simulink model "model_main4"  (R2023b)
settings: Solver=ode4  StartTime=0.0  StopTime=1000  FixedStep=dt  RelTol=1e-3
values from neighbouring files (symbols this model uses):
  dt = 0.01    [model_init.m]
  Iws = diag([1 1 1 1])*0.227    [model_init.m]
  m_tot = 3019.19    [model_init.m]
  Omega1_init = 1000*rpm2rad    (= 104.71975512)    [model_init.m]
  Omega2_init = 1000*rpm2rad    (= 104.71975512)    [model_init.m]
  Omega3_init = 1000*rpm2rad    (= 104.71975512)    [model_init.m]
  Omega4_init = 1000*rpm2rad    (= 104.71975512)    [model_init.m]
  qb0 = eul2quat(ag0','ZYX')'    [model_init.m]
  rad2rpm = 1/rpm2rad    (= 9.54929658551)    [model_init.m]
  RCS_F = 1.0    (= 1)    [model_init.m]
  RCS_Pos = [RCS1_POS , RCS2_POS , RCS3_POS , RCS4_POS ,            RCS5_POS , RCS6_POS , RCS7_POS , RCS8_POS ,            RCS9_POS , RCS10_POS, RCS11_POS, RCS12_POS,            RCS13_POS, RCS14_POS, RCS15_POS, RCS16_POS]    [model_init.m]
  RCS_PWM_Freq = 0.5    [model_init.m]
  RCS_Sampling_time = 0.01    [model_init.m]
  RCS_THR_vec = [RCS1_THR , RCS2_THR , RCS3_THR , RCS4_THR,                 RCS5_THR , RCS6_THR , RCS7_THR , RCS8_THR,                 RCS9_THR , RCS10_THR, RCS11_THR, RCS12_THR,                 RCS13_THR, RCS14_THR, RCS15_THR, RCS16_THR]    [model_init.m]
  REL_TS_POS_I_0 = TS_pos0 - SC_pos0    [model_init.m]
  REL_TS_VEL_I_0 = TS_vel0 - SC_vel0    [model_init.m]
  RW_As = [RW1_Axis,RW2_Axis,RW3_Axis,RW4_Axis]    [model_init.m]
  RW_Omegad_max = 4200*rpm2rad    (= 439.822971503)    [model_init.m]
  SC_Ib = [1257.52 -0.07285  -0.0345 ... (first row only)    [model_init.m]
  SC_state0 = kepel_statvec (SC_Kepler)    [model_init.m]
  TS_Ib = diag([1 1 1])    [model_init.m]
  TS_qb0 = angle2quat(deg2rad(0),deg2rad(0),deg2rad(0),'ZYX')'    [model_init.m]
  TS_state0 = kepel_statvec (TS_Kepler)    [model_init.m]
  TS_wb0 = deg2rad([0 0 0]')    [model_init.m]
  wb0 = [0 0 0]'    [model_init.m]
undefined symbols (not defined in the file or in its folder): norm_Ib, RCS_F_vec, RCS_pos, RW_Max_Speed, SS_Total_Mass, TC_Kepler
libraries: simulink x16, simulink_extras x13, sharedtransform x9, aerolibutil x8
(part 1 of 2)
settings Model: PacingRate=1.100000  Creator=yhj2019  LastModifiedBy=ASCL
settings DebuggingCC: UnderSpecifiedDimensionMsg=warning

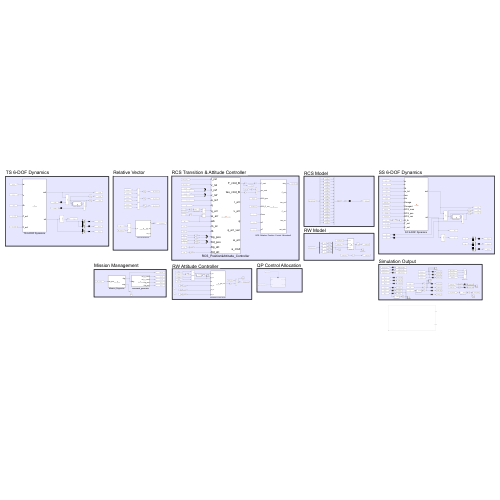
[thumbnail: Simulink's stored preview of the top-level diagram]
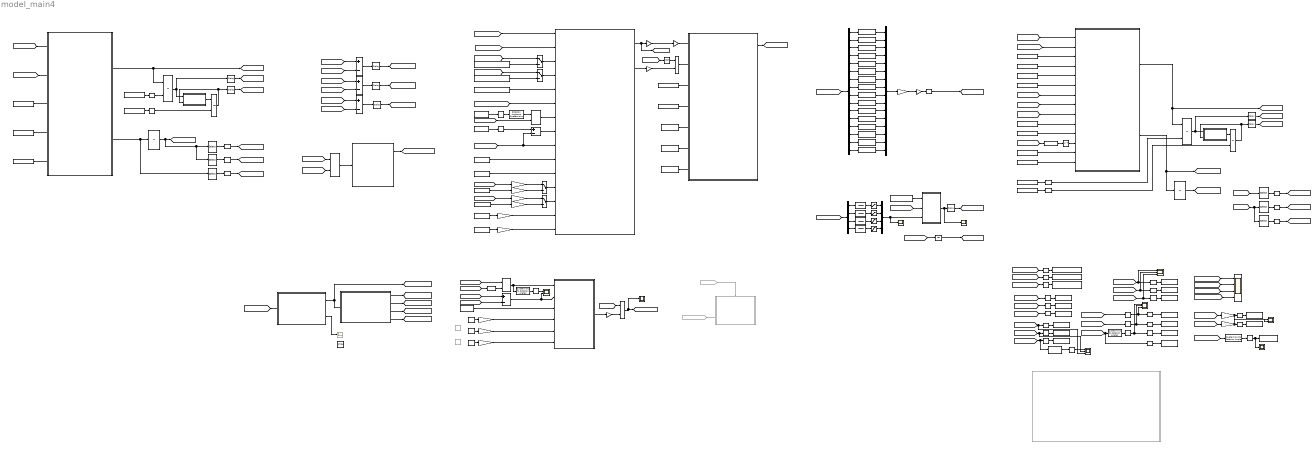
== system model_main4 ==
  note: TS 6-DOF Dynamics
  note: RW Model
  note: RW Attitude Controller
  note: RCS Model
  note: Simulation Output
  note: RCS Transition & Attitude Controller
  note: SS 6-DOF Dynamics
  note: Relative Vector
  note: Mission Management
  note: QP Control Allocation
  Add{,1..3,10} (5 alike) : Sum  Inputs=+-
  Constant : Constant  Value=0.3
  Constant1 : Constant  Value=17
  Constant{7,10,15,23,39,52} (6 alike) : Constant  Value=[0 0 0]'
  Constant11 : Constant  Value=RCS_Pos
  Constant12 : Constant  Value=RCS_THR_vec
  Constant13 : Constant  Value=m_tot
  Constant14 : Constant  Value=RW_Max_Speed
  Constant16 : Constant  Commented=on  Value=20
  Constant17 : Constant  Commented=on  Value=1000
  Constant18 : Constant  Value=200
  Constant19 : Constant  Value=10000
  Constant2 : Constant  Value=200
  Constant20 : Constant  Value=m_tot
  Constant21 : Constant  Value=0
  Constant3 : Constant  Value=2000
  Constant32 : Constant  Value=RW_As
  Constant36 : Constant  Value=TS_Ib
  Constant4 : Constant  Value=SC_Ib
  Constant40 : Constant  Value=TS_wb0
  Constant41 : Constant  Value=TS_qb0
  Constant49 : Constant  Value=[5.0 0 0]'
  Constant5 : Constant  Value=Iws
  Constant53 : Constant  Value=SC_Ib
  Constant55 : Constant
  Constant56 : Constant  Value=0.5
  Constant57 : Constant  Value=0.5
  Constant58 : Constant  Value=[0 0 0]
  Constant59 : Constant  Value=[0 0 0]
  Constant6 : Constant  Value=RW_As
  Constant60 : Constant  Value=RCS_Pos
  Constant61 : Constant  Value=RCS_THR_vec
  Constant8 : Constant  Value=wb0
  Constant9 : Constant  Value=qb0
  Degrees to Radians2 : simulink_extras/Transformations/Degrees to Radians
  Degrees to Radians3 : simulink_extras/Transformations/Degrees to Radians
  Demux : Demux  Outputs=16
  Demux1 : Demux
  Enabled Subsystem : Subsystem  Commented=on  TreatAsAtomicUnit=on
  From33 : From  Commented=on  GotoTag=mission_flag  TagVisibility=global
  From39 : From  Commented=on  GotoTag=RW_torque_cmd
  Gain{1,3,5..7,9,13,18,20} (9 alike) : Gain  Gain=norm_Ib
  Gain{2,10,12,23} (4 alike) : Gain
  Gain11 : Gain  Gain=rad2rpm
  Gain22 : Gain  Gain=-1
  Gain4 : Gain  Gain=RCS_F
  Gain8 : Gain  Gain=rad2rpm
  Get LOS Quaternion : MATLAB Function  TreatAsAtomicUnit=on
  Inetial to body : aerolibutil/Quaternion Rotation
  Integrator : Integrator  InitialConditionSource=external  InitialCondition=wb0
  Integrator2 : Integrator  InitialConditionSource=external  InitialCondition=wb0
  Integrator3 : Integrator  InitialCondition=[Omega1_init Omega2_init Omega3_init Omega4_init]'
  Integrator4 : Integrator  InitialConditionSource=external
  Integrator5 : Integrator  InitialCondition=TS_state0'
  Integrator7 : Integrator  InitialConditionSource=external
  Integrator8 : Integrator  InitialCondition=SC_state0'
  Los angle : Scope
  Manual Switch{,1,3..4} (4 alike) : ManualSwitch
  Mission_Supporter : MATLAB Function  TreatAsAtomicUnit=on
  Mux1 : Mux
  Mux2 : Mux  Inputs=16
  NOT : Logic  Operator=NOT  IconShape=distinctive  AllPortsSameDT=off  OutDataTypeStr=boolean
  PWM{,1..15} (16 alike) : simulink/Discontinuities/PWM  DisableCoverage=on  Period=RCS_PWM_Freq  InitialDelay=0  DisallowZeroDutyCycle=off  RunAtFixedTimeIntervals=on  SampleTime=RCS_Sampling_time
  Product : Product
  Product1 : Product
  Quaternion Inverse : aerolibutil/Quaternion Inverse
  Quaternion Multiplication1 : aerolibutil/Quaternion Multiplication
  Quaternion Multiplication4 : aerolibutil/Quaternion Multiplication
  Quaternion_Kinematics : MATLAB Function  TreatAsAtomicUnit=on
  Quaternion_Kinematics1 : MATLAB Function  TreatAsAtomicUnit=on
  Quaternions to Direction Cosine Matrix : sharedtransform/Quaternions to  Direction Cosine Matrix  aMode=aMode
      settings: LibrarySourceBlock=|
      | aerolibtransform2/Quaternions to
      | Direction Cosine Matrix
  Quaternions to Rotation Angles{,1..3} (4 alike) : sharedtransform/Quaternions to Rotation Angles  rotationOrder=ZYX  aMode=aMode
  RCS_Position&Attitude_Controller : MATLAB Function  TreatAsAtomicUnit=on
  RCS_Relative_Position_Control_Allocation2 : MATLAB Function  TreatAsAtomicUnit=on
  RW_torque_cmd : Scope
  Radians to Degrees{,1..5} (6 alike) : simulink_extras/Transformations/Radians to Degrees
  Rel transition / flag : Scope  NumInputPorts=4
  Reshape{,1..2,12..14,19..23} (11 alike) : Reshape  OutputDimensionality=Column vector (2-D)
  Reshape{3..11,15..18,24..28} (18 alike) : Reshape  OutputDimensionality=Row vector (2-D)
  Rotation Angles to Quaternions2 : sharedtransform/Rotation Angles to Quaternions  rotationOrder=ZYX  aMode=aMode
  SC 6-DOF Dynamics : MATLAB Function  TreatAsAtomicUnit=on
  SS Attitude Control wrt ECI : MATLAB Function  TreatAsAtomicUnit=on
  SS attitude : Scope  NumInputPorts=3
  SS transition : Scope  NumInputPorts=3
  Saturation{1..4} (4 alike) : Saturate  UpperLimit=RW_Omegad_max  LowerLimit=-RW_Omegad_max
  Scope : Scope  Commented=on
  Scope1 : Scope
  Scope2 : Scope
  Selector1 : Selector  InputPortWidth=6  IndexOptions=Index vector (dialog)  Indices=[1 2 3]  OutputSizes=1
  Selector2 : Selector  InputPortWidth=6  IndexOptions=Index vector (dialog)  Indices=[4 5 6]  OutputSizes=1
  Selector6 : Selector  InputPortWidth=6  IndexOptions=Index vector (dialog)  Indices=[1 2 3]  OutputSizes=1
  Selector7 : Selector  InputPortWidth=6  IndexOptions=Index vector (dialog)  Indices=[1 2 3]  OutputSizes=1
  Selector8 : Selector  InputPortWidth=6  IndexOptions=Index vector (dialog)  Indices=[4 5 6]  OutputSizes=1
  Selector9 : Selector  InputPortWidth=6  IndexOptions=Index vector (dialog)  Indices=[4 5 6]  OutputSizes=1
  Stop Simulation : Stop
  Subsystem : Subsystem  Commented=on
  TS 6-DOF Dynamics : MATLAB Function  TreatAsAtomicUnit=on
  Target attitude : Scope  NumInputPorts=3
  To Workspace : ToWorkspace  VariableName=SS_POS_I  SampleTime=-1
      settings: Save2DSignal=2-D array (concatenate along first dimension)
  To Workspace1 : ToWorkspace  VariableName=SS_VEL_I  SampleTime=-1
      settings: Save2DSignal=2-D array (concatenate along first dimension)
  To Workspace10 : ToWorkspace  VariableName=TS_VEL_I  SampleTime=-1
      settings: Save2DSignal=2-D array (concatenate along first dimension)
  To Workspace11 : ToWorkspace  VariableName=TS_ACC_I  SampleTime=-1
      settings: Save2DSignal=2-D array (concatenate along first dimension)
  To Workspace12 : ToWorkspace  VariableName=SS_q_b  SampleTime=-1
      settings: Save2DSignal=2-D array (concatenate along first dimension)
  To Workspace13 : ToWorkspace  VariableName=TS_wb  SampleTime=-1
      settings: Save2DSignal=2-D array (concatenate along first dimension)
  To Workspace14 : ToWorkspace  VariableName=wheel_rate  SampleTime=-1
      settings: Save2DSignal=2-D array (concatenate along first dimension)
  To Workspace15 : ToWorkspace  VariableName=TS_q  SampleTime=-1
      settings: Save2DSignal=2-D array (concatenate along first dimension)
  To Workspace16 : ToWorkspace  VariableName=TS_wd  SampleTime=-1
      settings: Save2DSignal=2-D array (concatenate along first dimension)
  To Workspace17 : ToWorkspace  VariableName=LoS_angle  SampleTime=-1
      settings: Save2DSignal=2-D array (concatenate along first dimension)
  To Workspace18 : ToWorkspace  VariableName=wheel_rated  SampleTime=-1
      settings: Save2DSignal=2-D array (concatenate along first dimension)
  To Workspace2 : ToWorkspace  VariableName=SS_ACC_I  SampleTime=-1
      settings: Save2DSignal=2-D array (concatenate along first dimension)
  To Workspace3 : ToWorkspace  VariableName=SS_wd_b  SampleTime=-1
      settings: Save2DSignal=2-D array (concatenate along first dimension)
  To Workspace4 : ToWorkspace  VariableName=SS_w_b  SampleTime=-1
      settings: Save2DSignal=2-D array (concatenate along first dimension)
  To Workspace5 : ToWorkspace  VariableName=SS_angle_I  SampleTime=-1
      settings: Save2DSignal=2-D array (concatenate along first dimension)
  To Workspace6 : ToWorkspace  VariableName=REL_TS_POS_I  SampleTime=-1
      settings: Save2DSignal=2-D array (concatenate along first dimension)
  To Workspace7 : ToWorkspace  VariableName=REL_TS_VEL_I  SampleTime=-1
      settings: Save2DSignal=2-D array (concatenate along first dimension)
  To Workspace8 : ToWorkspace  VariableName=REL_TS_ACC_I  SampleTime=-1
      settings: Save2DSignal=2-D array (concatenate along first dimension)
  To Workspace9 : ToWorkspace  VariableName=TS_POS_I  SampleTime=-1
      settings: Save2DSignal=2-D array (concatenate along first dimension)
  Transfer Fcn{,1..3} (4 alike) : TransferFcn  Numerator=[10]  Denominator=[1 10]
  Transport Delay1 : TransportDelay  DelayTime=dt  InitialOutput=qb0
  Transport Delay2 : TransportDelay  DelayTime=dt  InitialOutput=wb0
  Transport Delay3 : TransportDelay  DelayTime=dt  InitialOutput=[0 0 0]'
  Transport Delay4 : TransportDelay  DelayTime=dt  InitialOutput=REL_TS_VEL_I_0
  Transport Delay5 : TransportDelay  DelayTime=dt  InitialOutput=REL_TS_POS_I_0
  Transport Delay6 : TransportDelay  DelayTime=dt  InitialOutput=[0 0 0 0]'
  Transport Delay7 : TransportDelay  DelayTime=dt  InitialOutput=TS_qb0
  Transport Delay8 : TransportDelay  DelayTime=dt  InitialOutput=TS_wb0
  Transpose : Math  Operator=transpose
  attitude error : Scope  NumInputPorts=2
  command_generator : MATLAB Function  TreatAsAtomicUnit=on
  saturation : MATLAB Function  TreatAsAtomicUnit=on
  wheel rate : Scope  NumInputPorts=2
  tag scope: Kd_pos=global, Kp_pos=global, mission_flag=global, rel_p_cmd=global, rel_v_cmd=global
  wires:
  Reshape6/1 -> To Workspace/1
  Reshape7/1 -> To Workspace1/1
  Reshape8/1 -> To Workspace2/1
  [TS_p_I] -> Add/1
  [SS_p_I] -> Add/2
  [SS_v_I] -> Add1/2
  [TS_v_I] -> Add1/1
  [SS_a_I] -> Add2/2
  [TS_a_I] -> Add2/1
  Add/1 -> Transport Delay5/1
  Add1/1 -> Transport Delay4/1
  Add2/1 -> Transport Delay3/1
  Constant4/1 -> SC 6-DOF Dynamics/3(Ib)
  Constant5/1 -> SC 6-DOF Dynamics/5(Iws)
  SC 6-DOF Dynamics/1(wd) -> Integrator/1, [wd]
  [wb] -> SC 6-DOF Dynamics/1(w)
  Constant6/1 -> SC 6-DOF Dynamics/6(As)
  [Omega_mea] -> SC 6-DOF Dynamics/7(Omega)
  [Omegad_mea] -> SC 6-DOF Dynamics/8(Omegad)
  Quaternion_Kinematics/1(qd) -> Integrator7/1
  Constant8/1 -> Reshape19/1
  Constant9/1 -> Reshape20/1
  Quaternions to Rotation Angles/1 -> Radians to Degrees2/1
  [wd] -> Radians to Degrees/1
  [wb] -> Radians to Degrees1/1
  Radians to Degrees/1 -> SS attitude/3, Reshape9/1
  Radians to Degrees1/1 -> SS attitude/2, Reshape10/1
  Radians to Degrees2/1 -> SS attitude/1, Reshape11/1
  [q] -> Reshape3/1, Quaternions to Rotation Angles/1
  Constant10/1 -> SC 6-DOF Dynamics/14(F_ext)
  Constant13/1 -> SC 6-DOF Dynamics/4(m_tot)
  [q] -> Quaternions to Direction Cosine Matrix/1
  Quaternions to Direction Cosine Matrix/1 -> Transpose/1
  [SS_v_I] -> SS transition/2, Reshape7/1
  Transpose/1 -> SC 6-DOF Dynamics/12(R_Ib)
  Reshape9/1 -> To Workspace3/1
  Reshape10/1 -> To Workspace4/1
  Reshape11/1 -> To Workspace5/1
  SC 6-DOF Dynamics/2(xd) -> Integrator8/1, [xd]
  Integrator8/1 -> [x]
  Selector8/1 -> Reshape2/1
  Selector6/1 -> Reshape/1
  [xd] -> Selector8/1, Selector7/1
  [x] -> Selector6/1
  Selector7/1 -> Reshape1/1
  [x] -> SC 6-DOF Dynamics/2(x)
  Constant11/1 -> SC 6-DOF Dynamics/10(RCS_pos)
  Constant12/1 -> SC 6-DOF Dynamics/11(RCS_vec)
  Demux/1 -> PWM/1
  Demux/2 -> PWM1/1
  Demux/3 -> PWM2/1
  Demux/4 -> PWM3/1
  Demux/8 -> PWM7/1
  Demux/5 -> PWM4/1
  Demux/6 -> PWM5/1
  Demux/7 -> PWM6/1
  Demux/14 -> PWM13/1
  Demux/13 -> PWM12/1
  Demux/15 -> PWM14/1
  Demux/12 -> PWM11/1
  Demux/16 -> PWM15/1
  Demux/9 -> PWM8/1
  Demux/10 -> PWM9/1
  Demux/11 -> PWM10/1
  PWM/1 -> Mux2/1
  Mux2/1 -> Gain4/1
  PWM1/1 -> Mux2/2
  PWM2/1 -> Mux2/3
  PWM3/1 -> Mux2/4
  PWM4/1 -> Mux2/5
  PWM5/1 -> Mux2/6
  PWM6/1 -> Mux2/7
  PWM7/1 -> Mux2/8
  PWM8/1 -> Mux2/9
  PWM9/1 -> Mux2/10
  PWM10/1 -> Mux2/11
  PWM11/1 -> Mux2/12
  PWM12/1 -> Mux2/13
  PWM13/1 -> Mux2/14
  PWM14/1 -> Mux2/15
  PWM15/1 -> Mux2/16
  [RCS_mea] -> SC 6-DOF Dynamics/9(RCS_mea)
  Gain4/1 -> Gain12/1
  Reshape/1 -> [SS_p_I]
  Reshape1/1 -> [SS_v_I]
  Reshape2/1 -> [SS_a_I]
  [REL_TS_POS_I] -> Reshape16/1
  [REL_TS_VEL_I] -> Reshape17/1
  [REL_TS_ACC_I] -> Reshape18/1
  Reshape16/1 -> To Workspace6/1
  Reshape17/1 -> To Workspace7/1
  Reshape18/1 -> To Workspace8/1
  [REL_TS_POS_I] -> Rel transition / flag/1
  [REL_TS_VEL_I] -> Rel transition / flag/2
  [REL_TS_ACC_I] -> Rel transition / flag/3
  Constant32/1 -> SS Attitude Control wrt ECI/3(As)
  Get LOS Quaternion/1(q) -> [LoS_Quaternion]  "LOS quaternion"
  Add10/1 -> SS Attitude Control wrt ECI/2(w_err), attitude error/2
  [q] -> Inetial to body/1
  Inetial to body/1 -> Get LOS Quaternion/1(r_rel)
  SS Attitude Control wrt ECI/1(RW_cmd) -> Gain10/1
  [REL_TS_POS_I] -> Inetial to body/2
  Reshape19/1 -> Integrator/2
  Reshape20/1 -> Integrator7/2
  Gain12/1 -> Reshape14/1
  Demux1/1 -> Transfer Fcn/1
  Demux1/4 -> Transfer Fcn3/1
  Demux1/2 -> Transfer Fcn1/1
  Demux1/3 -> Transfer Fcn2/1
  Transfer Fcn/1 -> Saturation4/1
  Transfer Fcn1/1 -> Saturation1/1
  Transfer Fcn2/1 -> Saturation2/1
  Transfer Fcn3/1 -> Saturation3/1
  [Omegad_mea] -> Integrator3/1
  Integrator3/1 -> [Omega_mea]
  Integrator/1 -> Transport Delay2/1, Quaternion_Kinematics/1(w)
  Integrator7/1 -> Transport Delay1/1, Quaternion_Kinematics/2(q)
  [Omegad_mea] -> Gain8/1
  [Omega_mea] -> Gain11/1
  [RW_torque_cmd] -> Demux1/1
  saturation/1(res) -> RW_torque_cmd/1, Transport Delay6/1
  Saturation3/1 -> Mux1/4
  Saturation1/1 -> Mux1/2
  Saturation4/1 -> Mux1/1
  Saturation2/1 -> Mux1/3
  Mux1/1 -> Scope2/1, saturation/3(torque_cmd)
  [Omega_mea] -> saturation/2(Omega_mea)
  Constant14/1 -> saturation/1(max_speed)
  [SS_p_I] -> SS transition/1, Reshape6/1
  [SS_a_I] -> SS transition/3, Reshape8/1
  Reshape14/1 -> [RCS_mea]
  Transport Delay1/1 -> [q]
  Transport Delay2/1 -> [wb]
  Transport Delay3/1 -> [REL_TS_ACC_I]
  Transport Delay4/1 -> [REL_TS_VEL_I]
  Transport Delay5/1 -> [REL_TS_POS_I]
  Transport Delay6/1 -> [Omegad_mea]
  Transport Delay7/1 -> [TS_q]
  Integrator4/1 -> Quaternion_Kinematics1/2(q), Transport Delay7/1
  Constant39/1 -> TS 6-DOF Dynamics/4(T_ext)
  Integrator2/1 -> Quaternion_Kinematics1/1(w), Transport Delay8/1
  Constant41/1 -> Reshape13/1
  Transport Delay8/1 -> [TS_wb]
  Integrator5/1 -> Selector2/1, Selector1/1, [TS_x]
  Reshape13/1 -> Integrator4/2
  TS 6-DOF Dynamics/2(xd) -> Selector9/1, Integrator5/1
  [TS_x] -> TS 6-DOF Dynamics/2(x)
  Quaternion_Kinematics1/1(qd) -> Integrator4/1
  Constant15/1 -> TS 6-DOF Dynamics/5(F_ext)
  TS 6-DOF Dynamics/1(wd) -> [TS_wd], Integrator2/1
  Constant40/1 -> Reshape12/1
  [TS_wb] -> TS 6-DOF Dynamics/1(w)
  Constant36/1 -> TS 6-DOF Dynamics/3(Ib)
  Reshape12/1 -> Integrator2/2
  Reshape21/1 -> [TS_p_I]
  Selector1/1 -> Reshape21/1
  Reshape22/1 -> [TS_v_I]
  Reshape23/1 -> [TS_a_I]
  Selector9/1 -> Reshape23/1
  Selector2/1 -> Reshape22/1
  [TS_v_I] -> Reshape25/1
  [TS_a_I] -> Reshape26/1
  Reshape25/1 -> To Workspace10/1
  Reshape24/1 -> To Workspace9/1
  Reshape26/1 -> To Workspace11/1
  [TS_p_I] -> Reshape24/1
  Reshape3/1 -> To Workspace12/1
  Radians to Degrees4/1 -> To Workspace17/1, Los angle/1
  Quaternions to Rotation Angles3/1 -> Radians to Degrees4/1
  [TS_wd] -> Target attitude/3, Reshape4/1
  Reshape15/1 -> To Workspace15/1
  Reshape4/1 -> To Workspace16/1
  Reshape5/1 -> To Workspace13/1
  [TS_q] -> Quaternions to Rotation Angles1/1, Reshape15/1
  [TS_wb] -> Target attitude/2, Reshape5/1
  Gain7/1 -> RCS_Position&Attitude_Controller/14(Kp_att)
  RCS_Position&Attitude_Controller/2(tau_cmd_B) -> Gain23/1
  Constant20/1 -> RCS_Position&Attitude_Controller/10(m_sc)
  [REL_TS_POS_I] -> RCS_Position&Attitude_Controller/1(r_rel)
  Constant61/1 -> RCS_Relative_Position_Control_Allocation2/4(RCS_F_vec)
  Constant56/1 -> RCS_Relative_Position_Control_Allocation2/6(wF)
  Degrees to Radians3/1 -> Add3/1
  Constant1/1 -> Gain18/1
  [q] -> RCS_Position&Attitude_Controller/6("q ")
  [REL_TS_VEL_I] -> RCS_Position&Attitude_Controller/2(v_rel)
  RCS_Position&Attitude_Controller/1(F_cmd_B) -> [F_cmd_B], Gain2/1
  Constant59/1 -> Degrees to Radians3/1
  Constant58/1 -> Degrees to Radians2/1
  Gain3/1 -> RCS_Position&Attitude_Controller/15(Kd_att)
  Constant23/1 -> RCS_Position&Attitude_Controller/5(a_ref)
  RCS_Relative_Position_Control_Allocation2/1(duty) -> [RCS_PWPF_CMD]
  Constant55/1 -> RCS_Relative_Position_Control_Allocation2/5(Tmax)
  Constant2/1 -> Gain7/1
  Constant/1 -> Gain20/1
  Rotation Angles to Quaternions2/1 -> Quaternion Multiplication4/1
  Gain2/1 -> Gain22/1
  Degrees to Radians2/1 -> Rotation Angles to Quaternions2/1
  Quaternion Multiplication4/1 -> RCS_Position&Attitude_Controller/7(q_err)
  Constant57/1 -> RCS_Relative_Position_Control_Allocation2/7(wT)
  Constant60/1 -> RCS_Relative_Position_Control_Allocation2/3(RCS_pos)
  [LoS_Quaternion] -> Quaternion Multiplication4/2
  Gain22/1 -> RCS_Relative_Position_Control_Allocation2/1(F_cmd)
  [RCS_PWPF_CMD] -> Demux/1
  Constant53/1 -> RCS_Position&Attitude_Controller/11(Ib)
  [wb] -> Add3/2, RCS_Position&Attitude_Controller/9(wb)
  Constant3/1 -> Gain3/1
  Constant7/1 -> SC 6-DOF Dynamics/13(T_ext)
  [REL_TS_POS_I] -> Mission_Supporter/1(res_pos)
  Manual Switch1/1 -> RCS_Position&Attitude_Controller/4(v_ref)
  Manual Switch/1 -> RCS_Position&Attitude_Controller/3(r_ref)
  Constant52/1 -> Manual Switch1/2
  Constant49/1 -> Manual Switch/2
  Mission_Supporter/1(flag) -> command_generator/1(flag), [mission_flag]
  Manual Switch4/1 -> RCS_Position&Attitude_Controller/13(Kd_pos)
  Gain18/1 -> Manual Switch4/2
  Gain20/1 -> Manual Switch3/2
  command_generator/4(Kd_pos) -> [Kd_pos]
  command_generator/3(Kp_pos) -> [Kp_pos]
  command_generator/2(rel_v_cmd) -> [rel_v_cmd]
  command_generator/1(rel_p_cmd) -> [rel_p_cmd]
  [rel_v_cmd] -> Manual Switch1/1
  [rel_p_cmd] -> Manual Switch/1
  [mission_flag] -> Rel transition / flag/4
  Mission_Supporter/2(stop) -> Scope/1
  [Kp_pos] -> Gain1/1
  [Kd_pos] -> Gain5/1
  Gain5/1 -> Manual Switch4/1
  Gain1/1 -> Manual Switch3/1
  [LoS_Quaternion] -> Quaternions to Rotation Angles3/1
  Manual Switch3/1 -> RCS_Position&Attitude_Controller/12(Kp_pos)
  Gain23/1 -> Product/2
  Product/1 -> RCS_Relative_Position_Control_Allocation2/2(tau_cmd)
  Gain9/1 -> SS Attitude Control wrt ECI/5(Kd_rw)
  [mission_flag] -> Product1/1
  Gain10/1 -> Product1/2
  Product1/1 -> Scope1/1, [RW_torque_cmd]
  Gain6/1 -> SS Attitude Control wrt ECI/4(Kp_rw)
  Radians to Degrees3/1 -> Target attitude/1
  Quaternions to Rotation Angles1/1 -> Radians to Degrees3/1
  Add3/1 -> RCS_Position&Attitude_Controller/8("w_err ")
  Gain11/1 -> wheel rate/1, Reshape27/1
  Reshape27/1 -> To Workspace14/1
  Gain8/1 -> wheel rate/2, Reshape28/1
  Reshape28/1 -> To Workspace18/1
  From33/1 -> Enabled Subsystem/Enable
  [mission_flag] -> NOT/1
  NOT/1 -> Product/1
  From39/1 -> Enabled Subsystem/2(RCS_PD)
  [q] -> Quaternion Inverse/1
  Quaternion Inverse/1 -> Quaternion Multiplication1/2
  [TS_q] -> Quaternion Multiplication1/1
  [TS_wb] -> Add10/1
  [wb] -> Add10/2
  Quaternion Multiplication1/1 -> SS Attitude Control wrt ECI/1(q_err), Quaternions to Rotation Angles2/1
  Quaternions to Rotation Angles2/1 -> Radians to Degrees5/1
  Radians to Degrees5/1 -> attitude error/1
  Constant18/1 -> Gain6/1
  Constant19/1 -> Gain9/1
  Constant21/1 -> Gain13/1
  Gain13/1 -> SS Attitude Control wrt ECI/6(Ki_rw)

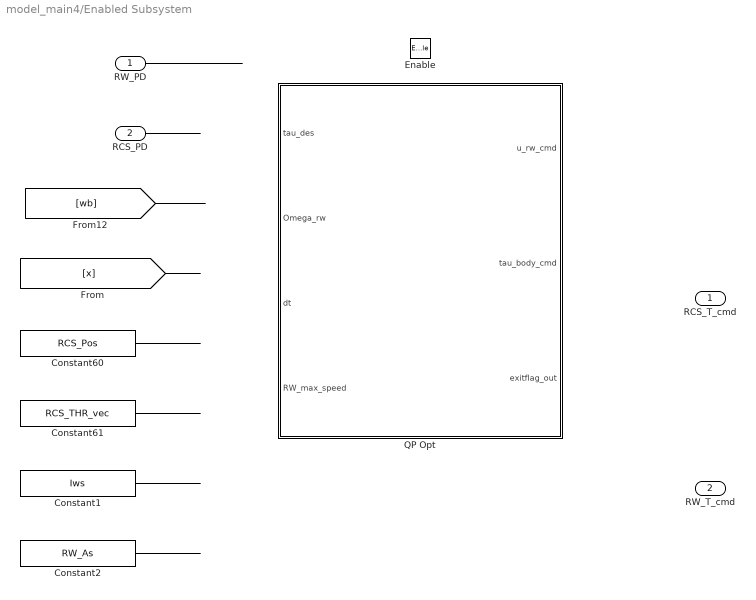
== system model_main4/Enabled Subsystem ==
  RW_PD : Inport
  RCS_PD : Inport  Port=2
  Enable : EnablePort
  Constant1 : Constant  Value=Iws
  Constant2 : Constant  Value=RW_As
  Constant60 : Constant  Value=RCS_Pos
  Constant61 : Constant  Value=RCS_THR_vec
  QP Opt : MATLAB Function  TreatAsAtomicUnit=on
  RCS_T_cmd : Outport
  RW_T_cmd : Outport  Port=2
  wires:
  RW_PD/1 -> ?
  RCS_PD/1 -> ?
  ? -> RCS_T_cmd/1
  ? -> RW_T_cmd/1
  [wb] -> ?
  [x] -> ?
  Constant60/1 -> ?
  Constant61/1 -> ?
  Constant1/1 -> ?
  Constant2/1 -> ?

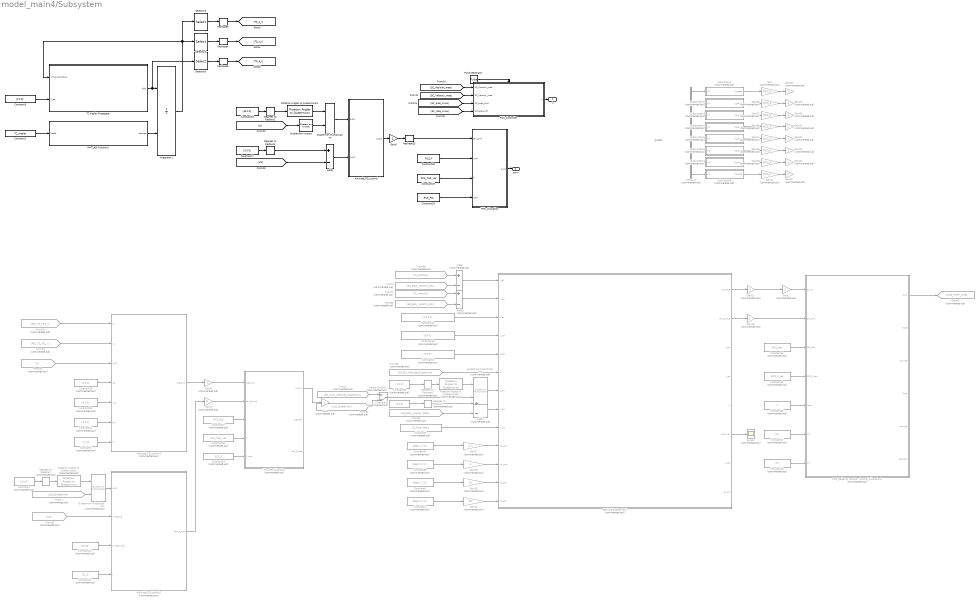
== system model_main4/Subsystem ==
  note: pwpfm
  Add12 : Sum  Commented=on  Inputs=+-
  Add15 : Sum  Commented=on  Inputs=+-
  Add3 : Sum  Inputs=+-
  Add6 : Sum  Commented=on  Inputs=+-
  Attitude_PD_control : MATLAB Function  TreatAsAtomicUnit=on
  Attitude_PD_control1 : MATLAB Function  Commented=on  TreatAsAtomicUnit=on
  Attitude_PD_control2 : MATLAB Function  Commented=on  TreatAsAtomicUnit=on
  Constant1 : Constant  Value=TC_Kepler
  Constant16 : Constant  Value=[45 0 0]
  Constant17 : Constant  Value=[0 0 0]
  Constant18 : Constant  Value=RCS_F
  Constant19 : Constant  Value=RCS_THR_vec
  Constant2 : Constant  Commented=on  Value=[0 0 0]
  Constant20 : Constant  Value=RCS_Pos
  Constant21 : Constant  Commented=on  Value=SC_Ib
  Constant{6,22,24..25,43} (5 alike) : Constant  Commented=on  Value=[0 0 0]'
  Constant26 : Constant  Commented=on  Value=[2 0 0]'
  Constant27 : Constant  Commented=on  Value=RCS_Pos
  Constant28 : Constant  Commented=on  Value=RCS_THR_vec
  Constant29 : Constant  Commented=on  Value=RCS_F
  Constant3 : Constant  Value=[0 0 0]'
  Constant{4,8,37..38} (4 alike) : Constant  Commented=on  Value=diag([1 1 1])
  Constant42 : Constant  Commented=on  Value=[1.5 0 0]'
  Constant44 : Constant  Commented=on  Value=RCS_pos
  Constant45 : Constant  Commented=on  Value=RCS_F_vec
  Constant46 : Constant  Commented=on
  Constant47 : Constant  Commented=on  Value=0.5
  Constant48 : Constant  Commented=on  Value=0.5
  Constant5 : Constant  Commented=on  Value=SS_Total_Mass
  Constant50 : Constant  Commented=on  Value=[0 0 0]
  Constant51 : Constant  Commented=on  Value=[0 0 0]
  Constant7 : Constant  Commented=on  Value=m_tot
  Degrees to Radians1 : simulink_extras/Transformations/Degrees to Radians
  Degrees to Radians2 : simulink_extras/Transformations/Degrees to Radians  Commented=on
  Degrees to Radians3 : simulink_extras/Transformations/Degrees to Radians
  Degrees to Radians6 : simulink_extras/Transformations/Degrees to Radians  Commented=on
  Degrees to Radians7 : simulink_extras/Transformations/Degrees to Radians  Commented=on
  Demux2 : Demux  Commented=on  Outputs=8
  From1 : From  Commented=on  GotoTag=LoS_Quaternion
  From2 : From  Commented=on  GotoTag=SS_LVLH_Attitude_Quaternion
  From3 : From  Commented=on  GotoTag=SS_Body_Position_ECI
  From30 : From  Commented=on  GotoTag=wb
  From31 : From  Commented=on  GotoTag=q
  From32 : From  Commented=on  GotoTag=REL_TS_POS_I
  From33 : From  Commented=on  GotoTag=REL_TS_VEL_I
  From39 : From  Commented=on  GotoTag=TS_Position
  From56 : From  Commented=on  GotoTag=SS_ECI_Attitude_Quaternion
  From61 : From  Commented=on  GotoTag=SS_Body_Angular_Rate
  From62 : From  Commented=on  GotoTag=LoS_Quaternion
  From69 : From  Commented=on  GotoTag=SS_Body_Velocity_ECI
  From72 : From  Commented=on  GotoTag=TS_Velocity
  Gain{,24..27,36..38} (8 alike) : Gain  Commented=on  Gain=RCS_F
  Gain1 : Gain  Commented=on  Gain=0
  Gain{6,13,28..35} (10 alike) : Gain  Commented=on  Gain=-1
  Gain14 : Gain  Commented=on  Gain=50
  Gain15 : Gain  Commented=on  Gain=10
  Gain{2,9,16,19} (4 alike) : Gain  Commented=on
  Gain17 : Gain  Commented=on  Gain=0.1
  Gain5 : Gain
  Get LOS Quaternion7 : MATLAB Function  Commented=on  TreatAsAtomicUnit=on
  Goto42 : Goto  Commented=on  GotoTag=RCS_PWPF_CMD
  Integrator1 : Integrator  InitialConditionSource=external  InitialCondition=[-7000 0 0 0 -9.175045 0 5233.5]'
  MATLAB Function1 : MATLAB Function  TreatAsAtomicUnit=on
  Manual Switch2 : ManualSwitch  Commented=on  CurrentSetting=0
  Pulse Generator : DiscretePulseGenerator  PulseType=Time based  Period=0.2  PulseWidth=50
  Quaternion Inverse : aerolibutil/Quaternion Inverse
  Quaternion Multiplication : aerolibutil/Quaternion Multiplication
  Quaternion Multiplication2 : aerolibutil/Quaternion Multiplication  Commented=on
  Quaternion Multiplication3 : aerolibutil/Quaternion Multiplication  Commented=on
  RCS_Controller : Subsystem
  RCS_Relative_Position_Control_Allocation1 : MATLAB Function  Commented=on  TreatAsAtomicUnit=on
  Reshape{3..5,15} (4 alike) : Reshape  OutputDimensionality=Column vector (2-D)
  Rotation Angles to Quaternions1 : sharedtransform/Rotation Angles to Quaternions  rotationOrder=ZYX  aMode=aMode
  Rotation Angles to Quaternions2 : sharedtransform/Rotation Angles to Quaternions  Commented=on  rotationOrder=ZYX  aMode=aMode
  Rotation Angles to Quaternions3 : sharedtransform/Rotation Angles to Quaternions  Commented=on  rotationOrder=ZYX  aMode=aMode
  Scope7 : Scope  Commented=on
  Selector3 : Selector  InputPortWidth=6  IndexOptions=Index vector (dialog)  Indices=[1 2 3]  OutputSizes=1
  Selector4 : Selector  InputPortWidth=6  IndexOptions=Index vector (dialog)  Indices=[4 5 6]  OutputSizes=1
  Selector5 : Selector  InputPortWidth=6  IndexOptions=Index vector (dialog)  Indices=[4 5 6]  OutputSizes=1
  Subsystem1 : Subsystem  Commented=on
  Subsystem2 : Subsystem  Commented=on
  Subsystem3 : Subsystem  Commented=on
  Subsystem4 : Subsystem  Commented=on
  Subsystem5 : Subsystem  Commented=on
  Subsystem6 : Subsystem  Commented=on
  Subsystem7 : Subsystem  Commented=on
  Subsystem8 : Subsystem  Commented=on
  TC Kepler Propagate : MATLAB Function  TreatAsAtomicUnit=on
  THR_Allocation : MATLAB Function  TreatAsAtomicUnit=on
  Thruster Allocation : MATLAB Function  Commented=on  TreatAsAtomicUnit=on
  u : Outport
  pwm : Outport  Port=2
  wires:
  Reshape15/1 -> THR_Allocation/1(tau_cmd)
  Selector4/1 -> Reshape4/1
  TC Kepler Propagate/1(dfdt) -> Selector5/1, Integrator1/1
  Pulse Generator/1 -> RCS_Controller/Trigger
  [SC_quat_LVLH] -> RCS_Controller/3(SC_quat_LVLH)
  Constant16/1 -> Degrees to Radians1/1
  Quaternion Multiplication/1 -> Attitude_PD_control/1(q_err)
  [q] -> Quaternion Inverse/1
  Selector5/1 -> Reshape5/1
  Gain5/1 -> Reshape15/1
  [SC_rate_LVLH] -> RCS_Controller/4(SC_rate_LVLH)
  Constant1/1 -> MATLAB Function1/1(kepel)
  Attitude_PD_control/1(u_torq) -> Gain5/1
  [SC_Position_mea] -> RCS_Controller/1(SC_Position_mea)
  Constant17/1 -> Degrees to Radians3/1
  Integrator1/1 -> Selector3/1, TC Kepler Propagate/1(initial_condition), Selector4/1
  Constant19/1 -> THR_Allocation/3(f)
  MATLAB Function1/1(statvec) -> Integrator1/2
  Constant20/1 -> THR_Allocation/4(r_thr)
  Reshape5/1 -> [TS_a_I]
  Constant3/1 -> TC Kepler Propagate/2(F_eci)
  [SC_Velocity_mea] -> RCS_Controller/2(SC_Velocity_mea)
  Degrees to Radians1/1 -> Rotation Angles to Quaternions1/1
  Rotation Angles to Quaternions1/1 -> Quaternion Multiplication/1
  [wb] -> Add3/2
  Constant18/1 -> THR_Allocation/2(F_on)
  Selector3/1 -> Reshape3/1
  Reshape4/1 -> [TS_v_I]
  Add3/1 -> Attitude_PD_control/2(w_err)
  Reshape3/1 -> [TS_p_I]
  Degrees to Radians3/1 -> Add3/1
  Quaternion Inverse/1 -> Quaternion Multiplication/2
  RCS_Controller/1(u) -> u/1
  THR_Allocation/1(pwm) -> pwm/1
  Get LOS Quaternion7/1(F_cmd_B) -> Gain13/1
  Add12/1 -> Get LOS Quaternion7/8("w_err ")
  Constant7/1 -> Attitude_PD_control1/7(m)
  Degrees to Radians6/1 -> Rotation Angles to Quaternions3/1
  Constant8/1 -> Gain15/1
  Quaternion Multiplication2/1 -> Attitude_PD_control2/1(q_err)
  From2/1 -> Manual Switch2/1
  Quaternion Multiplication3/1 -> Get LOS Quaternion7/7(q_err)
  Gain13/1 -> Gain2/1
  Gain14/1 -> Get LOS Quaternion7/13(Kd_att)
  Rotation Angles to Quaternions3/1 -> Quaternion Multiplication3/1
  Manual Switch2/1 -> Quaternion Multiplication3/2
  Gain2/1 -> RCS_Relative_Position_Control_Allocation1/1(F_cmd)
  Add6/1 -> Get LOS Quaternion7/1(r_rel)
  From31/1 -> Attitude_PD_control1/3(q_IB)
  Constant22/1 -> Attitude_PD_control2/3(omega_d_B)
  From39/1 -> Add6/1
  From3/1 -> Add6/2
  Constant27/1 -> Thruster Allocation/3(r)
  Constant28/1 -> Thruster Allocation/4(d)
  Constant2/1 -> Degrees to Radians2/1
  Attitude_PD_control2/1(tau_B_cmd) -> Gain1/1
  Constant46/1 -> RCS_Relative_Position_Control_Allocation1/5(Tmax)
  RCS_Relative_Position_Control_Allocation1/1(duty) -> Goto42/1
  Constant6/1 -> Get LOS Quaternion7/5(a_ref)
  Get LOS Quaternion7/2(tau_cmd_B) -> Gain19/1
  Constant51/1 -> Degrees to Radians7/1
  From32/1 -> Attitude_PD_control1/1(r_I)
  Constant37/1 -> Gain17/1
  Constant47/1 -> RCS_Relative_Position_Control_Allocation1/6(wF)
  From30/1 -> Attitude_PD_control2/2(omega_B)
  Constant43/1 -> Get LOS Quaternion7/4(v_ref)
  Constant29/1 -> Thruster Allocation/5(F_max)
  Constant26/1 -> Attitude_PD_control1/4(r_d)
  Rotation Angles to Quaternions2/1 -> Quaternion Multiplication2/1
  Constant50/1 -> Degrees to Radians6/1
  From1/1 -> Quaternion Multiplication2/2
  From62/1 -> Manual Switch2/2
  Constant21/1 -> Attitude_PD_control2/4(J)
  Constant44/1 -> RCS_Relative_Position_Control_Allocation1/3(RCS_pos)
  From72/1 -> Add15/1
  Gain16/1 -> Get LOS Quaternion7/11(Kd_pos)
  Degrees to Radians2/1 -> Rotation Angles to Quaternions2/1
  Gain6/1 -> Thruster Allocation/1(F_B_cmd)
  Get LOS Quaternion7/6(q_err_vec) -> Scope7/1
  From56/1 -> Get LOS Quaternion7/6("q ")
  From69/1 -> Add15/2
  Attitude_PD_control1/1(F_B_cmd) -> Gain6/1
  Thruster Allocation/1(u_pwm) -> Gain9/1
  Gain1/1 -> Thruster Allocation/2(tau_B_cmd)
  Degrees to Radians7/1 -> Add12/1
  Gain19/1 -> RCS_Relative_Position_Control_Allocation1/2(tau_cmd)
  From61/1 -> Add12/2
  Constant5/1 -> Get LOS Quaternion7/9(m_sc)
  Constant25/1 -> Attitude_PD_control1/5(v_d)
  Constant24/1 -> Attitude_PD_control1/6(a_d)
  From33/1 -> Attitude_PD_control1/2(v_I)
  Constant38/1 -> Gain16/1
  Constant48/1 -> RCS_Relative_Position_Control_Allocation1/7(wT)
  Constant4/1 -> Gain14/1
  Constant45/1 -> RCS_Relative_Position_Control_Allocation1/4(RCS_F_vec)
  Gain15/1 -> Get LOS Quaternion7/12(Kp_att)
  Gain17/1 -> Get LOS Quaternion7/10(Kp_pos)
  Constant42/1 -> Get LOS Quaternion7/3(r_ref)
  Add15/1 -> Get LOS Quaternion7/2(v_rel)
  Demux2/4 -> Subsystem4/1(In1)
  Demux2/5 -> Subsystem5/1(In1)
  Subsystem2/1(F_gated) -> Gain36/1
  Gain26/1 -> Gain34/1
  Gain38/1 -> Gain31/1
  Demux2/7 -> Subsystem7/1(In1)
  Gain27/1 -> Gain35/1
  Subsystem6/1(F_gated) -> Gain25/1
  Demux2/3 -> Subsystem3/1(In1)
  Subsystem3/1(F_gated) -> Gain37/1
  Demux2/6 -> Subsystem6/1(In1)
  Subsystem7/1(F_gated) -> Gain26/1
  Gain36/1 -> Gain29/1
  Gain24/1 -> Gain32/1
  Demux2/8 -> Subsystem8/1(In1)
  Subsystem1/1(F_gated) -> Gain/1
  Gain37/1 -> Gain30/1
  Subsystem4/1(F_gated) -> Gain38/1
  Gain/1 -> Gain28/1
  Subsystem8/1(F_gated) -> Gain27/1
  Gain25/1 -> Gain33/1
  Demux2/2 -> Subsystem2/1(In1)
  Subsystem5/1(F_gated) -> Gain24/1
  Demux2/1 -> Subsystem1/1(In1)

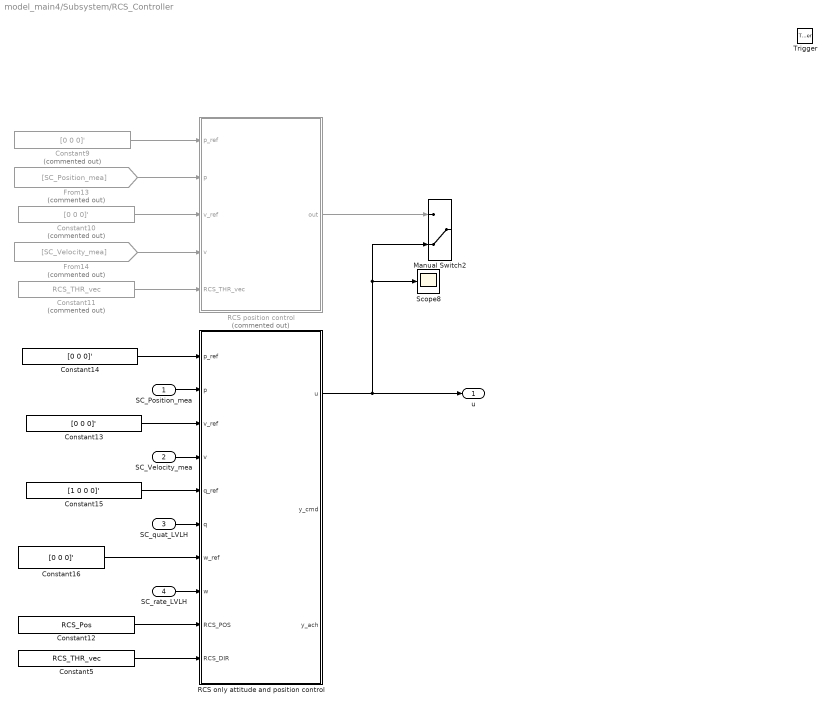
== system model_main4/Subsystem/RCS_Controller ==
  SC_Position_mea : Inport
  SC_Velocity_mea : Inport  Port=2
  SC_quat_LVLH : Inport  Port=3
  SC_rate_LVLH : Inport  Port=4
  Trigger : TriggerPort  TriggerType=either  VariantControl=(inherit)  PortDimensions=1
  Constant10 : Constant  Commented=on  Value=[0 0 0]'
  Constant11 : Constant  Commented=on  Value=RCS_THR_vec
  Constant12 : Constant  Value=RCS_Pos
  Constant13 : Constant  Value=[0 0 0]'
  Constant14 : Constant  Value=[0 0 0]'
  Constant15 : Constant  Value=[1 0 0 0]'
  Constant16 : Constant  Value=[0 0 0]'
  Constant5 : Constant  Value=RCS_THR_vec
  Constant9 : Constant  Commented=on  Value=[0 0 0]'
  From13 : From  Commented=on  GotoTag=SC_Position_mea  TagVisibility=global
  From14 : From  Commented=on  GotoTag=SC_Velocity_mea  TagVisibility=global
  Manual Switch2 : ManualSwitch  CurrentSetting=0
  RCS only attitude and position control : MATLAB Function  TreatAsAtomicUnit=on
  RCS position control : MATLAB Function  Commented=on  TreatAsAtomicUnit=on
  Scope8 : Scope
  u : Outport
  wires:
  Constant5/1 -> RCS only attitude and position control/10(RCS_DIR)
  SC_quat_LVLH/1 -> RCS only attitude and position control/6(q)
  Constant12/1 -> RCS only attitude and position control/9(RCS_POS)
  SC_rate_LVLH/1 -> RCS only attitude and position control/8(w)
  SC_Velocity_mea/1 -> RCS only attitude and position control/4(v)
  From13/1 -> RCS position control/2(p)
  RCS only attitude and position control/1(u) -> Manual Switch2/2, Scope8/1, u/1
  Constant13/1 -> RCS only attitude and position control/3(v_ref)
  Constant15/1 -> RCS only attitude and position control/5(q_ref)
  RCS position control/1(out) -> Manual Switch2/1
  Constant16/1 -> RCS only attitude and position control/7(w_ref)
  Constant10/1 -> RCS position control/3(v_ref)
  Constant9/1 -> RCS position control/1(p_ref)
  Constant11/1 -> RCS position control/5(RCS_THR_vec)
  SC_Position_mea/1 -> RCS only attitude and position control/2(p)
  Constant14/1 -> RCS only attitude and position control/1(p_ref)
  From14/1 -> RCS position control/4(v)

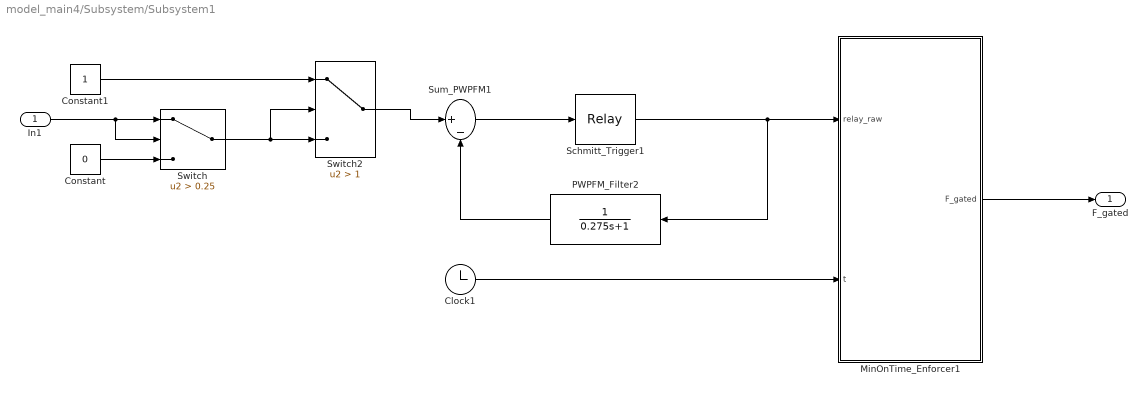
== system model_main4/Subsystem/Subsystem1 ==
  In1 : Inport
  Clock1 : Clock
  Constant : Constant  Value=0
  Constant1 : Constant
  MinOnTime_Enforcer1 : MATLAB Function  TreatAsAtomicUnit=on
  PWPFM_Filter2 : TransferFcn  Numerator=1  Denominator=[0.275 1]
  Schmitt_Trigger1 : Relay  OnSwitchValue=0.127  OffSwitchValue=-0.127
  Sum_PWPFM1 : Sum  Inputs=|+-
  Switch : Switch  Criteria=u2 > Threshold  Threshold=0.25  SaturateOnIntegerOverflow=off  InputSameDT=off
  Switch2 : Switch  Criteria=u2 > Threshold  Threshold=1  SaturateOnIntegerOverflow=off  InputSameDT=off
  F_gated : Outport
  wires:
  Schmitt_Trigger1/1 -> MinOnTime_Enforcer1/1(relay_raw), PWPFM_Filter2/1
  PWPFM_Filter2/1 -> Sum_PWPFM1/2
  Sum_PWPFM1/1 -> Schmitt_Trigger1/1
  MinOnTime_Enforcer1/1(F_gated) -> F_gated/1
  Clock1/1 -> MinOnTime_Enforcer1/2(t)
  Switch2/1 -> Sum_PWPFM1/1
  Constant1/1 -> Switch2/1
  Switch/1 -> Switch2/3, Switch2/2
  Constant/1 -> Switch/3
  In1/1 -> Switch/1, Switch/2

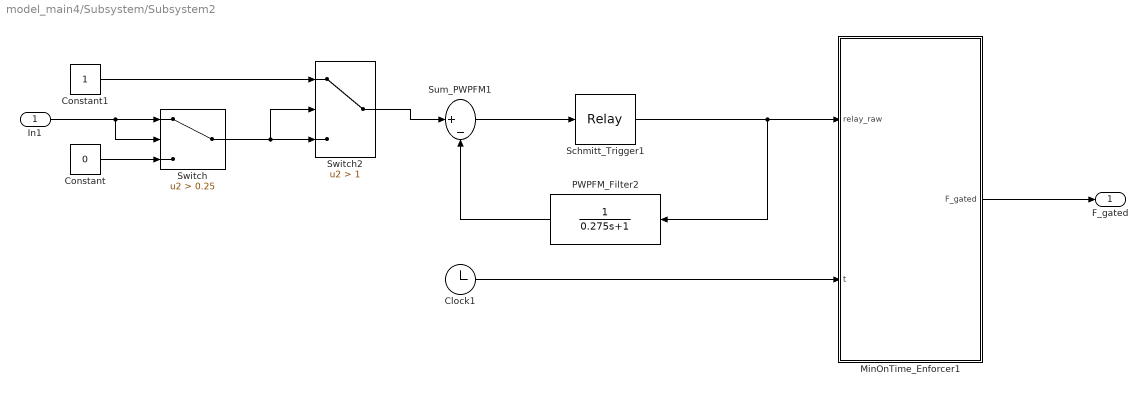
== system model_main4/Subsystem/Subsystem2 ==
  In1 : Inport
  Clock1 : Clock
  Constant : Constant  Value=0
  Constant1 : Constant
  MinOnTime_Enforcer1 : MATLAB Function  TreatAsAtomicUnit=on
  PWPFM_Filter2 : TransferFcn  Numerator=1  Denominator=[0.275 1]
  Schmitt_Trigger1 : Relay  OnSwitchValue=0.127  OffSwitchValue=-0.127
  Sum_PWPFM1 : Sum  Inputs=|+-
  Switch : Switch  Criteria=u2 > Threshold  Threshold=0.25  SaturateOnIntegerOverflow=off  InputSameDT=off
  Switch2 : Switch  Criteria=u2 > Threshold  Threshold=1  SaturateOnIntegerOverflow=off  InputSameDT=off
  F_gated : Outport
  wires:
  Schmitt_Trigger1/1 -> MinOnTime_Enforcer1/1(relay_raw), PWPFM_Filter2/1
  PWPFM_Filter2/1 -> Sum_PWPFM1/2
  Sum_PWPFM1/1 -> Schmitt_Trigger1/1
  MinOnTime_Enforcer1/1(F_gated) -> F_gated/1
  Clock1/1 -> MinOnTime_Enforcer1/2(t)
  Switch2/1 -> Sum_PWPFM1/1
  Constant1/1 -> Switch2/1
  Switch/1 -> Switch2/3, Switch2/2
  Constant/1 -> Switch/3
  In1/1 -> Switch/1, Switch/2

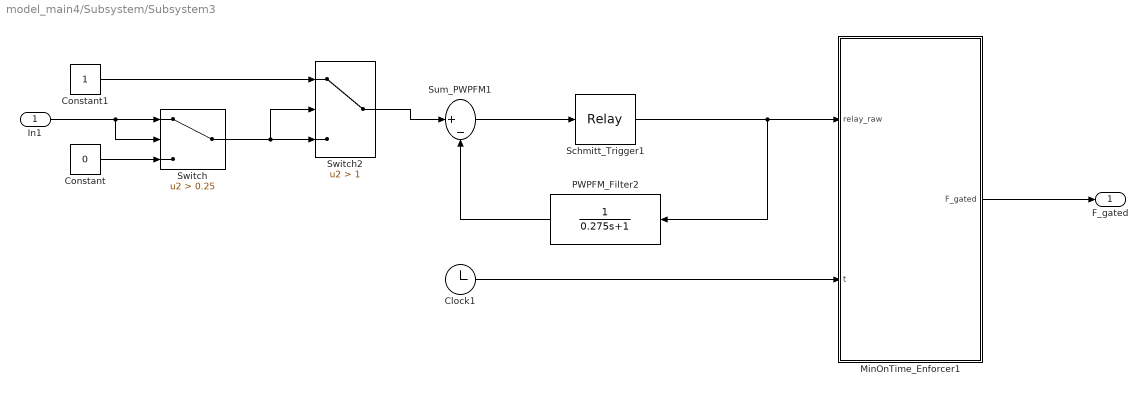
== system model_main4/Subsystem/Subsystem3 ==
  In1 : Inport
  Clock1 : Clock
  Constant : Constant  Value=0
  Constant1 : Constant
  MinOnTime_Enforcer1 : MATLAB Function  TreatAsAtomicUnit=on
  PWPFM_Filter2 : TransferFcn  Numerator=1  Denominator=[0.275 1]
  Schmitt_Trigger1 : Relay  OnSwitchValue=0.127  OffSwitchValue=-0.127
  Sum_PWPFM1 : Sum  Inputs=|+-
  Switch : Switch  Criteria=u2 > Threshold  Threshold=0.25  SaturateOnIntegerOverflow=off  InputSameDT=off
  Switch2 : Switch  Criteria=u2 > Threshold  Threshold=1  SaturateOnIntegerOverflow=off  InputSameDT=off
  F_gated : Outport
  wires:
  Schmitt_Trigger1/1 -> MinOnTime_Enforcer1/1(relay_raw), PWPFM_Filter2/1
  PWPFM_Filter2/1 -> Sum_PWPFM1/2
  Sum_PWPFM1/1 -> Schmitt_Trigger1/1
  MinOnTime_Enforcer1/1(F_gated) -> F_gated/1
  Clock1/1 -> MinOnTime_Enforcer1/2(t)
  Switch2/1 -> Sum_PWPFM1/1
  Constant1/1 -> Switch2/1
  Switch/1 -> Switch2/3, Switch2/2
  Constant/1 -> Switch/3
  In1/1 -> Switch/1, Switch/2

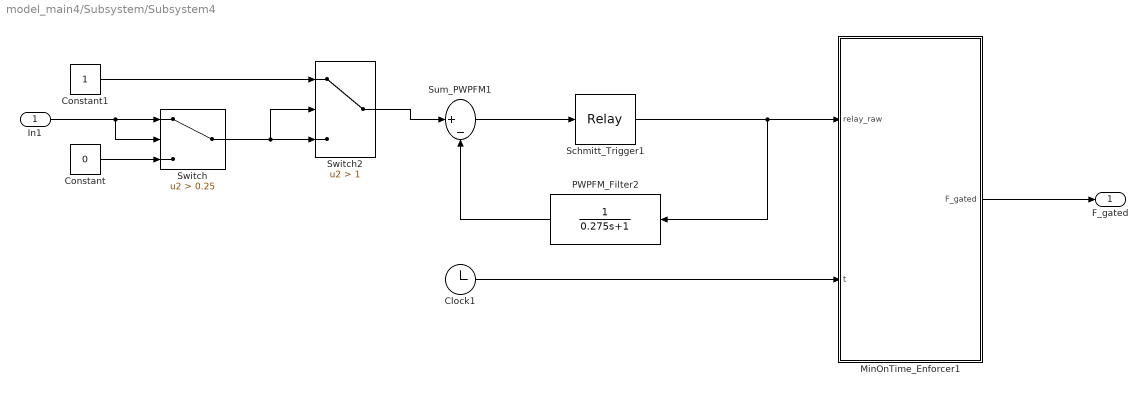
== system model_main4/Subsystem/Subsystem4 ==
  In1 : Inport
  Clock1 : Clock
  Constant : Constant  Value=0
  Constant1 : Constant
  MinOnTime_Enforcer1 : MATLAB Function  TreatAsAtomicUnit=on
  PWPFM_Filter2 : TransferFcn  Numerator=1  Denominator=[0.275 1]
  Schmitt_Trigger1 : Relay  OnSwitchValue=0.127  OffSwitchValue=-0.127
  Sum_PWPFM1 : Sum  Inputs=|+-
  Switch : Switch  Criteria=u2 > Threshold  Threshold=0.25  SaturateOnIntegerOverflow=off  InputSameDT=off
  Switch2 : Switch  Criteria=u2 > Threshold  Threshold=1  SaturateOnIntegerOverflow=off  InputSameDT=off
  F_gated : Outport
  wires:
  Schmitt_Trigger1/1 -> MinOnTime_Enforcer1/1(relay_raw), PWPFM_Filter2/1
  PWPFM_Filter2/1 -> Sum_PWPFM1/2
  Sum_PWPFM1/1 -> Schmitt_Trigger1/1
  MinOnTime_Enforcer1/1(F_gated) -> F_gated/1
  Clock1/1 -> MinOnTime_Enforcer1/2(t)
  Switch2/1 -> Sum_PWPFM1/1
  Constant1/1 -> Switch2/1
  Switch/1 -> Switch2/3, Switch2/2
  Constant/1 -> Switch/3
  In1/1 -> Switch/1, Switch/2

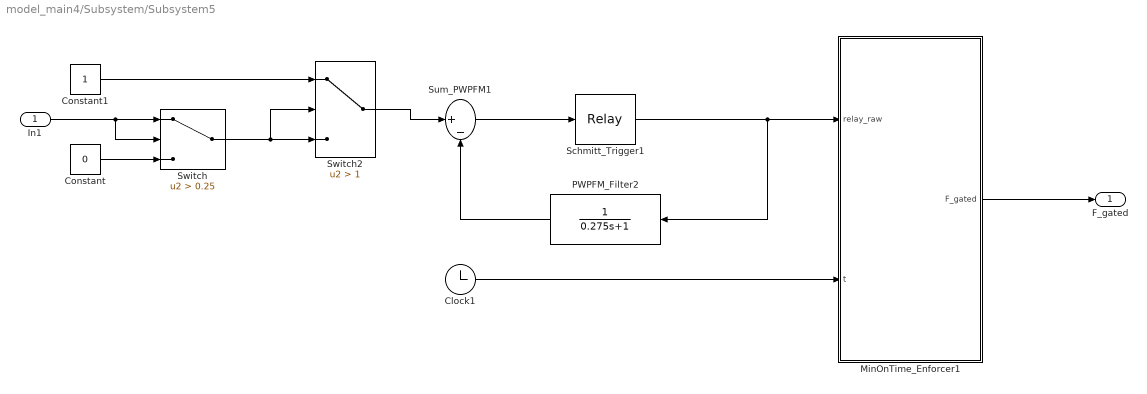
== system model_main4/Subsystem/Subsystem5 ==
  In1 : Inport
  Clock1 : Clock
  Constant : Constant  Value=0
  Constant1 : Constant
  MinOnTime_Enforcer1 : MATLAB Function  TreatAsAtomicUnit=on
  PWPFM_Filter2 : TransferFcn  Numerator=1  Denominator=[0.275 1]
  Schmitt_Trigger1 : Relay  OnSwitchValue=0.127  OffSwitchValue=-0.127
  Sum_PWPFM1 : Sum  Inputs=|+-
  Switch : Switch  Criteria=u2 > Threshold  Threshold=0.25  SaturateOnIntegerOverflow=off  InputSameDT=off
  Switch2 : Switch  Criteria=u2 > Threshold  Threshold=1  SaturateOnIntegerOverflow=off  InputSameDT=off
  F_gated : Outport
  wires:
  Schmitt_Trigger1/1 -> MinOnTime_Enforcer1/1(relay_raw), PWPFM_Filter2/1
  PWPFM_Filter2/1 -> Sum_PWPFM1/2
  Sum_PWPFM1/1 -> Schmitt_Trigger1/1
  MinOnTime_Enforcer1/1(F_gated) -> F_gated/1
  Clock1/1 -> MinOnTime_Enforcer1/2(t)
  Switch2/1 -> Sum_PWPFM1/1
  Constant1/1 -> Switch2/1
  Switch/1 -> Switch2/3, Switch2/2
  Constant/1 -> Switch/3
  In1/1 -> Switch/1, Switch/2

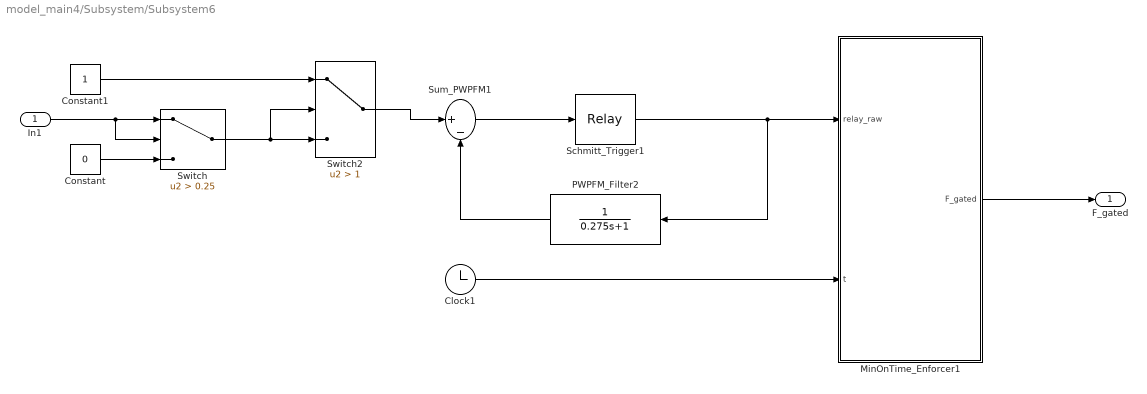
== system model_main4/Subsystem/Subsystem6 ==
  In1 : Inport
  Clock1 : Clock
  Constant : Constant  Value=0
  Constant1 : Constant
  MinOnTime_Enforcer1 : MATLAB Function  TreatAsAtomicUnit=on
  PWPFM_Filter2 : TransferFcn  Numerator=1  Denominator=[0.275 1]
  Schmitt_Trigger1 : Relay  OnSwitchValue=0.127  OffSwitchValue=-0.127
  Sum_PWPFM1 : Sum  Inputs=|+-
  Switch : Switch  Criteria=u2 > Threshold  Threshold=0.25  SaturateOnIntegerOverflow=off  InputSameDT=off
  Switch2 : Switch  Criteria=u2 > Threshold  Threshold=1  SaturateOnIntegerOverflow=off  InputSameDT=off
  F_gated : Outport
  wires:
  Schmitt_Trigger1/1 -> MinOnTime_Enforcer1/1(relay_raw), PWPFM_Filter2/1
  PWPFM_Filter2/1 -> Sum_PWPFM1/2
  Sum_PWPFM1/1 -> Schmitt_Trigger1/1
  MinOnTime_Enforcer1/1(F_gated) -> F_gated/1
  Clock1/1 -> MinOnTime_Enforcer1/2(t)
  Switch2/1 -> Sum_PWPFM1/1
  Constant1/1 -> Switch2/1
  Switch/1 -> Switch2/3, Switch2/2
  Constant/1 -> Switch/3
  In1/1 -> Switch/1, Switch/2

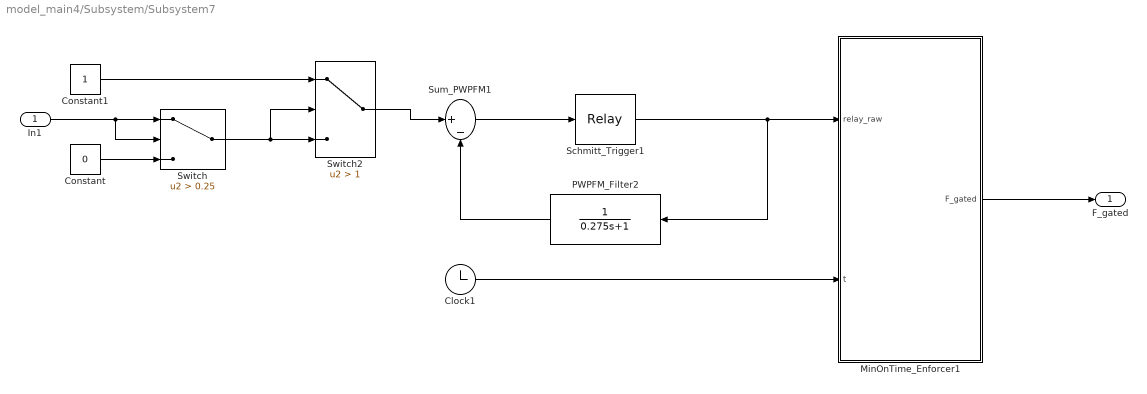
== system model_main4/Subsystem/Subsystem7 ==
  In1 : Inport
  Clock1 : Clock
  Constant : Constant  Value=0
  Constant1 : Constant
  MinOnTime_Enforcer1 : MATLAB Function  TreatAsAtomicUnit=on
  PWPFM_Filter2 : TransferFcn  Numerator=1  Denominator=[0.275 1]
  Schmitt_Trigger1 : Relay  OnSwitchValue=0.127  OffSwitchValue=-0.127
  Sum_PWPFM1 : Sum  Inputs=|+-
  Switch : Switch  Criteria=u2 > Threshold  Threshold=0.25  SaturateOnIntegerOverflow=off  InputSameDT=off
  Switch2 : Switch  Criteria=u2 > Threshold  Threshold=1  SaturateOnIntegerOverflow=off  InputSameDT=off
  F_gated : Outport
  wires:
  Schmitt_Trigger1/1 -> MinOnTime_Enforcer1/1(relay_raw), PWPFM_Filter2/1
  PWPFM_Filter2/1 -> Sum_PWPFM1/2
  Sum_PWPFM1/1 -> Schmitt_Trigger1/1
  MinOnTime_Enforcer1/1(F_gated) -> F_gated/1
  Clock1/1 -> MinOnTime_Enforcer1/2(t)
  Switch2/1 -> Sum_PWPFM1/1
  Constant1/1 -> Switch2/1
  Switch/1 -> Switch2/3, Switch2/2
  Constant/1 -> Switch/3
  In1/1 -> Switch/1, Switch/2

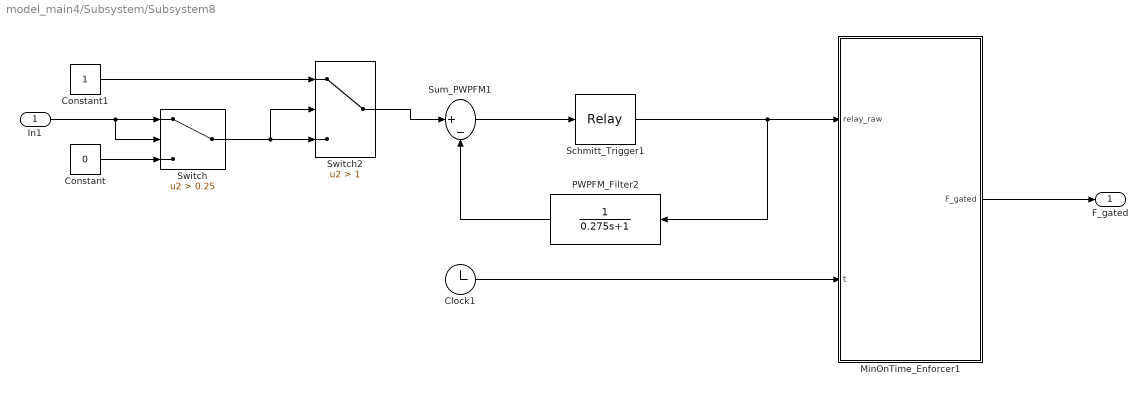
== system model_main4/Subsystem/Subsystem8 ==
  In1 : Inport
  Clock1 : Clock
  Constant : Constant  Value=0
  Constant1 : Constant
  MinOnTime_Enforcer1 : MATLAB Function  TreatAsAtomicUnit=on
  PWPFM_Filter2 : TransferFcn  Numerator=1  Denominator=[0.275 1]
  Schmitt_Trigger1 : Relay  OnSwitchValue=0.127  OffSwitchValue=-0.127
  Sum_PWPFM1 : Sum  Inputs=|+-
  Switch : Switch  Criteria=u2 > Threshold  Threshold=0.25  SaturateOnIntegerOverflow=off  InputSameDT=off
  Switch2 : Switch  Criteria=u2 > Threshold  Threshold=1  SaturateOnIntegerOverflow=off  InputSameDT=off
  F_gated : Outport
  wires:
  Schmitt_Trigger1/1 -> MinOnTime_Enforcer1/1(relay_raw), PWPFM_Filter2/1
  PWPFM_Filter2/1 -> Sum_PWPFM1/2
  Sum_PWPFM1/1 -> Schmitt_Trigger1/1
  MinOnTime_Enforcer1/1(F_gated) -> F_gated/1
  Clock1/1 -> MinOnTime_Enforcer1/2(t)
  Switch2/1 -> Sum_PWPFM1/1
  Constant1/1 -> Switch2/1
  Switch/1 -> Switch2/3, Switch2/2
  Constant/1 -> Switch/3
  In1/1 -> Switch/1, Switch/2

== matlab function model_main4/Subsystem/RCS_Controller/RCS only attitude and position control ==
  data: p_ref input; u output; p input; v_ref input; v input; q_ref input; q input; w_ref input; w input; RCS_POS input; RCS_DIR input; y_cmd output; y_ach output
function [u, y_cmd, y_ach] = fcn( ...
                                  p_ref, p, v_ref, v, ...          % position control
                                  q_ref, q, w_ref, w, ...          % attitude control (quat + body rates)
                                  RCS_POS, RCS_DIR)                % thruster geometry
%#codegen
% p, v : 3x1 [m], [m/s]
% q_ref, q : 4x1 quaternion (scalar-first: [qw qx qy qz]')
% w_ref, w : 3x1 [rad/s] (body frame)
% RCS_POS : 3xN position vectors of thrusters wrt CoM [m]
% RCS_DIR : 3xN thrust direction unit vectors [N/A] in body frame
% u : Nx1 thrust commands [N]

% ====== Parameters ======
Tmax = 22;       % [N]
m    = 2000;     % [kg]

% Translational PD gains
Kp_p = 2 * diag([1 1 1]);
Kd_p = 4 * diag([1 1 1]);

% Attitude PD gains (원하시면 사용하신 K1,K2 그대로 넣으셔도 됩니다)
Kq = 0.5 * diag([1 1 1]);    % quaternion-vector part gain
Kw = 2  * diag([1 1 1]);    % angular-rate gain

% (선택) 힘/토크 가중치: 단위/스케일 차이 때문에 보통 넣는 걸 권장합니다.
wF   = 1.0;    % force weight
wTau = 1.0;    % torque weight (필요 시 크게/작게 조정)

% ====== 1) Translation: PD -> F_cmd ======
e_p = p_ref - p;
e_v = v_ref - v;

a_cmd = Kp_p*e_p + Kd_p*e_v;
F_cmd = m * a_cmd;              % 3x1

% ====== 2) Attitude: quaternion error + rate error -> Tau_cmd ======
qe = quat_err_scalar_first(q_ref, q);     % q_err = q_ref ⊗ conj(q)
% 쿼터니언 언와인딩 방지(연속성)
if qe(1) < 0
    qe = -qe;
end
qe_v = qe(2:4);

we = w - w_ref;                 % body rate error (원하시면 w_ref-w 로 바꾸셔도 됨)

% 기본적인 PD 토크(부호는 시스템 정의에 맞게 조정 가능)
Tau_cmd = -(Kq*qe_v + Kw*we);    % 3x1

% ====== 3) Build 6xN allocation matrix B ======
N = size(RCS_DIR, 2);

B = zeros(6, N);
for i = 1:N
    ti = RCS_DIR(:, i);          % 3x1
    ri = RCS_POS(:, i);          % 3x1
    B(1:3, i) = ti;
    B(4:6, i) = cross(ri, ti);
end

% ====== 4) Stack command y = [F; Tau] and solve allocation ======
y_cmd = [wF*F_cmd; wTau*Tau_cmd];      % 6x1
Bw    = [wF*B(1:3,:); wTau*B(4:6,:)];  % weighted B

% 간단 대안: pinv + clip + active-set 반복(툴박스 없이 가능)
u = rcs_allocate_pinv_clip_iter(Bw, y_cmd, Tmax);

y_ach = B*u;    % achieved (unweighted, physical)

end

% ===== Helper: iterative clipped pseudo-inverse allocation =====
function u = rcs_allocate_pinv_clip_iter(B, y, Tmax)
%#codegen
N = size(B,2);

% 초기 해
u = pinv(B) * y;

% active-set 반복: 0 또는 Tmax에 걸린 추력기는 고정하고 나머지만 재해결
MAX_IT = 10;
for k = 1:MAX_IT
    u_prev = u;

    % bounds 적용
    u = max(u, 0);
    u = min(u, Tmax);

    % 자유 변수 마스크
    free = (u > 1e-9) & (u < Tmax - 1e-9);

    if ~any(free)
        break;
    end

    % 고정된 변수 기여를 빼고, 자유 변수만 재계산
    y_res = y - B(:, ~free) * u(~free);
    Bf    = B(:, free);

    uf = pinv(Bf) * y_res;

    u(free) = uf;

    % 수렴 체크
    if norm(u - u_prev) < 1e-6
        break;
    end
end
end

% ===== Helper: quaternion error (scalar-first) =====
function qe = quat_err_scalar_first(q_ref, q)
%#codegen
% qe = q_ref ⊗ conj(q)
qc = [q(1); -q(2); -q(3); -q(4)];

qe = quat_mul_scalar_first(q_ref, qc);
end

function q = quat_mul_scalar_first(q1, q2)
%#codegen
w1=q1(1); x1=q1(2); y1=q1(3); z1=q1(4);
w2=q2(1); x2=q2(2); y2=q2(3); z2=q2(4);

q = [ ...
    w1*w2 - x1*x2 - y1*y2 - z1*z2; ...
    w1*x2 + x1*w2 + y1*z2 - z1*y2; ...
    w1*y2 - x1*z2 + y1*w2 + z1*x2; ...
    w1*z2 + x1*y2 - y1*x2 + z1*w2  ...
    ];
end

== matlab function model_main4/Subsystem/RCS_Controller/RCS position control ==
  data: p_ref input; out output; p input; v_ref input; v input; RCS_THR_vec input
function out = fcn(p_ref, p, v_ref, v, RCS_THR_vec)
% ====== 파라미터 ======
Tmax   = 22;       % [N]
m = 2000;
% pwmMax = 65535;    % 예: 16-bit
% pwmMin = 0;        % 필요하면 최소 구동값 넣기
Kp = 20*diag([1 1 1]);
Kd = 40*diag([1 1 1]);
% ====== 1) PD -> F_cmd ======
e_p = p_ref - p;
e_v = v_ref - v;

a_cmd = Kp*e_p + Kd*e_v;
F_cmd = m * a_cmd;

% ====== 2) Allocation ======
% [u, F_ach] = rcs_allocate_lsqlin(F_cmd, RCS_THR_vec, Tmax); % toolbox 권장
[u, F_ach] = rcs_allocate_pinv_clip(F_cmd, RCS_THR_vec, Tmax); % 간단 대안

% ====== 3) PWM ======
% pwm = thrust_to_pwm(u, Tmax, pwmMax, pwmMin);
out = u./1;
% (디버그)
% disp("F_cmd  = " + mat2str(F_cmd',4))
% disp("F_ach  = " + mat2str(F_ach',4))
% disp("u(N)   = " + mat2str(u',4))
% disp("pwm    = " + mat2str(pwm',4))

end

function [u, F_ach] = rcs_allocate_pinv_clip(F_cmd, RCS_THR_vec, Tmax)
    B = RCS_THR_vec;     % 3xN
    u = pinv(B) * F_cmd; % unconstrained

    % Thruster는 보통 단방향(0~Tmax)이므로 음수는 0으로
    u = max(u, 0);
    u = min(u, Tmax);

    F_ach = B*u;
end


function pwm = thrust_to_pwm(u, Tmax, pwmMax, pwmMin)
    % u: Nx1 thrust command [N]
    % pwmMax: 예) 65535 또는 255
    % pwmMin: (선택) 밸브/드라이버가 실제로 열리는 최소 duty가 있으면 반영

    duty = u(:) / Tmax;          % 0~1
    duty = max(0, min(1, duty));

    if nargin >= 4 && pwmMin > 0
        % duty>0인 경우에만 최소 구동 듀티 적용(데드존)
        duty(duty>0) = max(duty(duty>0), pwmMin/pwmMax);
    end

    pwm = round(duty * pwmMax);
end
